simulink model "sistema_electrico"  (R2013a)
settings: Solver=ode45  StartTime=0.0  StopTime=40  MaxStep=0.5  RelTol=1e-3
settings Model: Creator=Said  LastModifiedBy=Said
settings DataIOCC: LimitDataPoints=off

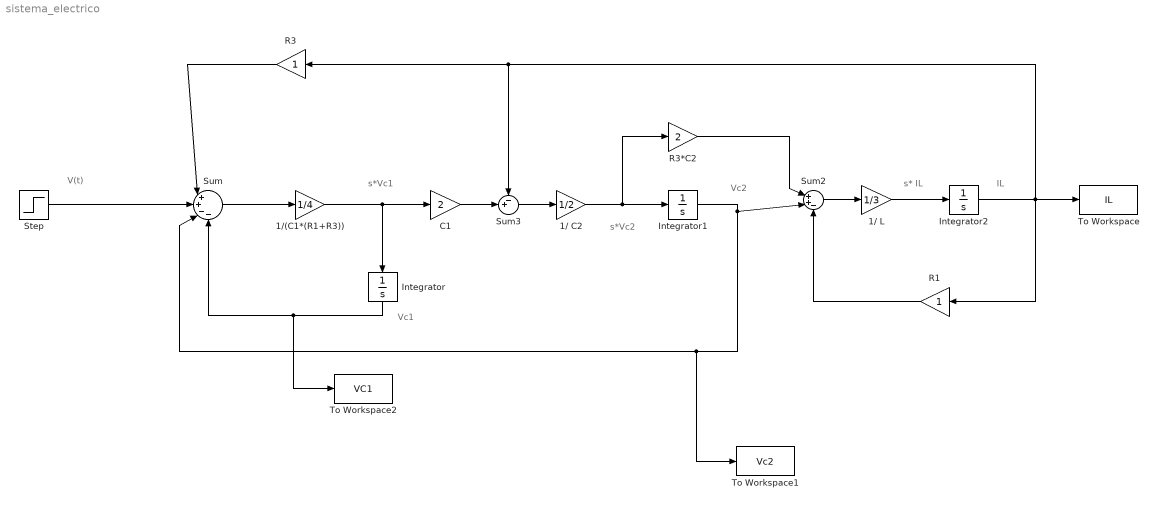
== system sistema_electrico ==
  note: V(t)
  note: Vc1
  note: s*Vc1
  note: s*Vc2
  note: Vc2
  note: s* IL
  note: IL
  1/ C2 : Gain  Gain=1/2
  1/ L : Gain  Gain=1/3
  1/(C1*(R1+R3)) : Gain  Gain=1/4
  C1 : Gain  Gain=2
  Integrator : Integrator
  Integrator1 : Integrator
  Integrator2 : Integrator
  R1 : Gain
  R3 : Gain
  R3*C2 : Gain  Gain=2
  Step : Step  Before=3  After=4  SampleTime=0
  Sum : Sum  Inputs=|++--
  Sum2 : Sum  Inputs=|++-
  Sum3 : Sum  Inputs=-+|
  To Workspace : ToWorkspace  VariableName=IL  SampleTime=-1
  To Workspace1 : ToWorkspace  VariableName=Vc2  SampleTime=-1
  To Workspace2 : ToWorkspace  VariableName=VC1  SampleTime=-1
  wires:
  Sum/1 -> 1/(C1*(R1+R3))/1
  1/(C1*(R1+R3))/1 -> C1/1, Integrator/1
  Integrator/1 -> To Workspace2/1, Sum/4
  1/ C2/1 -> R3*C2/1, Integrator1/1
  R3*C2/1 -> Sum2/1
  Integrator1/1 -> To Workspace1/1, Sum/3, Sum2/2
  Sum2/1 -> 1/ L/1
  1/ L/1 -> Integrator2/1
  C1/1 -> Sum3/2
  Sum3/1 -> 1/ C2/1
  R3/1 -> Sum/1
  Integrator2/1 -> To Workspace/1, Sum3/1, R3/1, R1/1
  R1/1 -> Sum2/3
  Step/1 -> Sum/2
